simulink model "model_openloop"  (R2021a)
settings: Solver=VariableStepAuto  StartTime=0.0  StopTime=100  RelTol=1e-3  EnableMultiTasking=on
values from neighbouring files (symbols this model uses):
  BE_rpm2kgps = BE_rpm2mmps*BE_mm2cc*BE_cc2g/1000    (= 5.30929158457e-05)    [constants.m]
  Cnst = [jf1,jf2,jf3,jh1,jh2,jh3,mf1,mf2,mf3,mh,mp,rbx,m,g,kd0,kd,kl0,kl,km0,km,k1,k2]    [constants.m]
  mb0 = 1    [constants.m]
  MM_MM_rpms2mpss = MM_rpms2mmpss*MM_mm2mm/1000    (= 2.27603686636e-05)    [constants.m]
  RM_costet2z = 2    [constants.m]
  RM_rpm2radps = 2*pi/60    (= 0.10471975512)    [constants.m]
  RM_sintet2y = 2    [constants.m]
  rpx0 = 0    [constants.m]
  rpy0 = 0    [constants.m]
  rpz0 = 0.05    [constants.m]
settings Model: Creator=Zein  LastModifiedBy=zein
settings SolverCC: AlgebraicLoopSolver=TrustRegion
settings DataIOCC: ReturnWorkspaceOutputs=off
settings OptimizationCC: LifeSpan=inf
settings DebuggingCC: SFUnexpectedBacktrackingDiag=warning  SFNoUnconditionalDefaultTransitionDiag=warning  SFMachineParentedDataDiag=warning  ArithmeticOperatorsInVariantConditions=warning
settings SFSimCC: SimUseLocalCustomCode=off  CustomCodeUndefinedFunction=UseInterfaceOnly
settings RTWCC: RTWUseLocalCustomCode=off
settings CodeAppCC: StateflowObjectComments=on
settings GRTTargetCC: TargetLangStandard=C89/C90 (ANSI)
settings ConfigComp: CovMetricSettings=dw  CovSaveCumulativeToWorkspaceVar=on  CovSaveSingleToWorkspaceVar=on  CovExternalEMLEnable=off

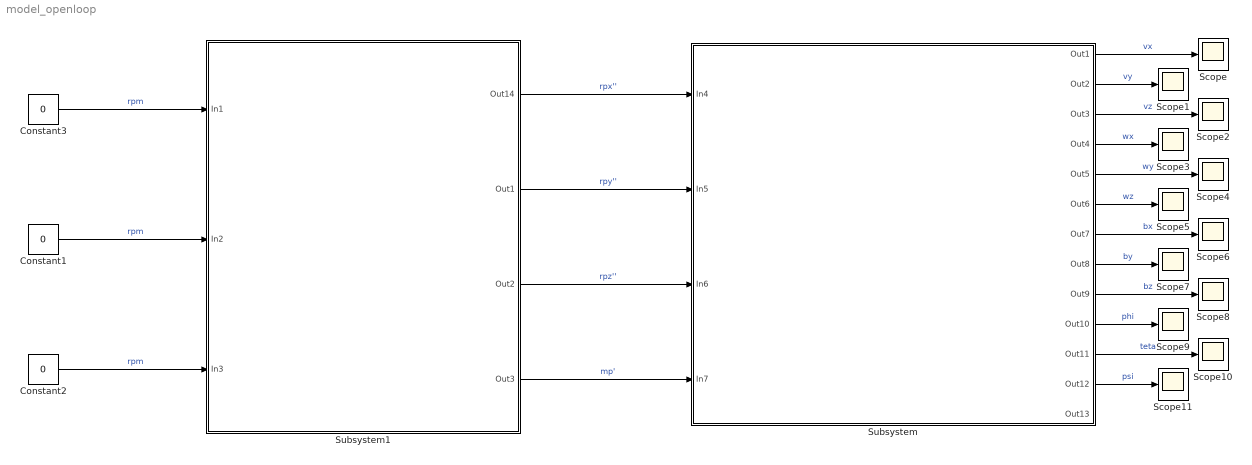
== system model_openloop ==
  Constant1 : Constant  Value=0
  Constant2 : Constant  Value=0
  Constant3 : Constant  Value=0
  Scope{,1..11} (12 alike) : Scope
  Subsystem : Subsystem
  Subsystem1 : Subsystem
  wires:
  Constant1/1 -> Subsystem1/2(In2)  "rpm"
  Constant2/1 -> Subsystem1/3(In3)  "rpm"
  Subsystem1/1(Out14) -> Subsystem/1(In4)  "rpx''"
  Subsystem1/2(Out1) -> Subsystem/2(In5)  "rpy''"
  Subsystem1/3(Out2) -> Subsystem/3(In6)  "rpz''"
  Subsystem1/4(Out3) -> Subsystem/4(In7)  "mp'"
  Subsystem/1(Out1) -> Scope/1  "vx"
  Subsystem/2(Out2) -> Scope1/1  "vy"
  Subsystem/4(Out4) -> Scope3/1  "wx"
  Subsystem/3(Out3) -> Scope2/1  "vz"
  Subsystem/6(Out6) -> Scope5/1  "wz"
  Subsystem/5(Out5) -> Scope4/1  "wy"
  Subsystem/7(Out7) -> Scope6/1  "bx"
  Subsystem/10(Out10) -> Scope9/1  "phi"
  Subsystem/9(Out9) -> Scope8/1  "bz"
  Subsystem/12(Out12) -> Scope11/1  "psi"
  Subsystem/11(Out11) -> Scope10/1  "teta"
  Subsystem/8(Out8) -> Scope7/1  "by"
  Constant3/1 -> Subsystem1/1(In1)  "rpm"

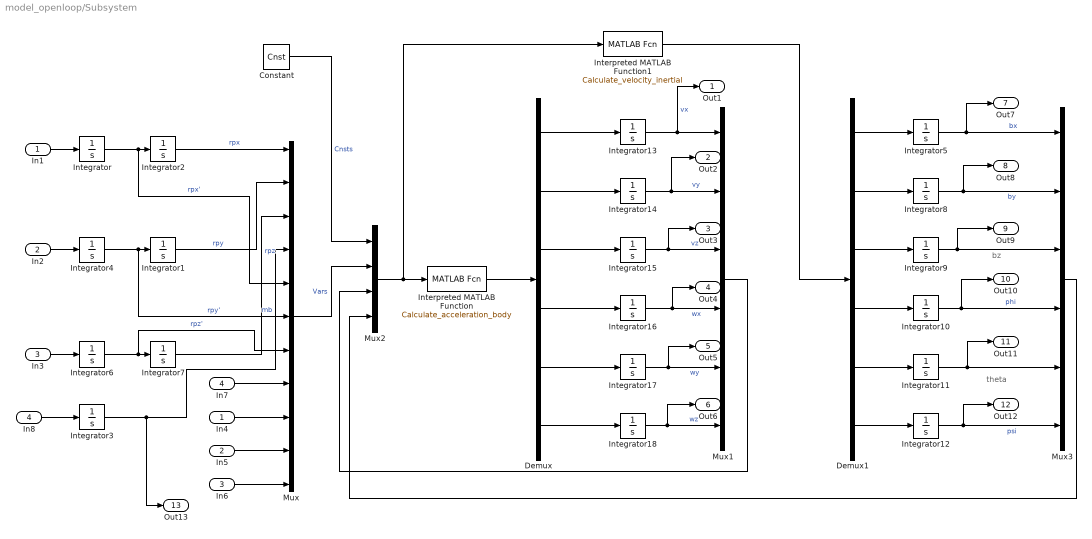
== system model_openloop/Subsystem ==
  note: theta
  note: bz
  In4 : Inport
  In5 : Inport  Port=2
  In6 : Inport  Port=3
  In7 : Inport  Port=4
  Constant : Constant  Value=Cnst
  Demux : Demux  Outputs=6
  Demux1 : Demux  Outputs=6
  In1 : InportShadow
  In2 : InportShadow  Port=2
  In3 : InportShadow  Port=3
  In8 : InportShadow  Port=4
  Integrator{,4..6,8..18} (15 alike) : Integrator
  Integrator1 : Integrator  InitialCondition=rpy0
  Integrator2 : Integrator  InitialCondition=rpx0
  Integrator3 : Integrator  InitialCondition=mb0
  Integrator7 : Integrator  InitialCondition=rpz0
  Interpreted MATLAB Function : MATLABFcn  MATLABFcn=Calculate_acceleration_body  OutputDimensions=6
  Interpreted MATLAB Function1 : MATLABFcn  MATLABFcn=Calculate_velocity_inertial  OutputDimensions=6  Output1D=off
  Mux : Mux  Inputs=11
  Mux1 : Mux  Inputs=6
  Mux2 : Mux
  Mux3 : Mux  Inputs=6
  Out1 : Outport
  Out2 : Outport  Port=2
  Out3 : Outport  Port=3
  Out4 : Outport  Port=4
  Out5 : Outport  Port=5
  Out6 : Outport  Port=6
  Out7 : Outport  Port=7
  Out8 : Outport  Port=8
  Out9 : Outport  Port=9
  Out10 : Outport  Port=10
  Out11 : Outport  Port=11
  Out12 : Outport  Port=12
  Out13 : Outport  Port=13
  wires:
  Demux1/2 -> Integrator8/1
  Integrator9/1 -> Out9/1, Mux3/3
  Integrator8/1 -> Out8/1, Mux3/2  "by"
  Integrator18/1 -> Out6/1, Mux1/6  "wz"
  Integrator16/1 -> Out4/1, Mux1/4  "wx"
  Demux/3 -> Integrator15/1
  Integrator15/1 -> Out3/1, Mux1/3  "vz"
  Interpreted MATLAB Function/1 -> Demux/1
  Demux/5 -> Integrator17/1
  Demux1/5 -> Integrator11/1
  Demux/2 -> Integrator14/1
  Mux3/1 -> Mux2/4
  Interpreted MATLAB Function1/1 -> Demux1/1
  Demux1/3 -> Integrator9/1
  Constant/1 -> Mux2/1  "Cnsts"
  Demux/6 -> Integrator18/1
  Demux/4 -> Integrator16/1
  Demux1/6 -> Integrator12/1
  Demux/1 -> Integrator13/1
  Integrator14/1 -> Out2/1, Mux1/2  "vy"
  Integrator17/1 -> Out5/1, Mux1/5  "wy"
  Demux1/4 -> Integrator10/1
  Integrator13/1 -> Out1/1, Mux1/1  "vx"
  Integrator12/1 -> Out12/1, Mux3/6  "psi"
  Integrator11/1 -> Out11/1, Mux3/5
  Integrator5/1 -> Out7/1, Mux3/1  "bx"
  Integrator10/1 -> Out10/1, Mux3/4  "phi"
  Demux1/1 -> Integrator5/1
  Mux2/1 -> Interpreted MATLAB Function1/1, Interpreted MATLAB Function/1
  Mux1/1 -> Mux2/3
  Integrator1/1 -> Mux/2  "rpy"
  Integrator/1 -> Mux/5, Integrator2/1  "rpx'"
  In6/1 -> Mux/11
  In5/1 -> Mux/10
  Integrator6/1 -> Mux/7, Integrator7/1  "rpz'"
  Integrator4/1 -> Mux/6, Integrator1/1  "rpy'"
  Integrator3/1 -> Out13/1, Mux/4  "mb"
  Integrator2/1 -> Mux/1  "rpx"
  Integrator7/1 -> Mux/3  "rpz"
  In7/1 -> Mux/8
  Mux/1 -> Mux2/2  "Vars"
  In4/1 -> Mux/9
  In1/1 -> Integrator/1
  In2/1 -> Integrator4/1
  In3/1 -> Integrator6/1
  In8/1 -> Integrator3/1

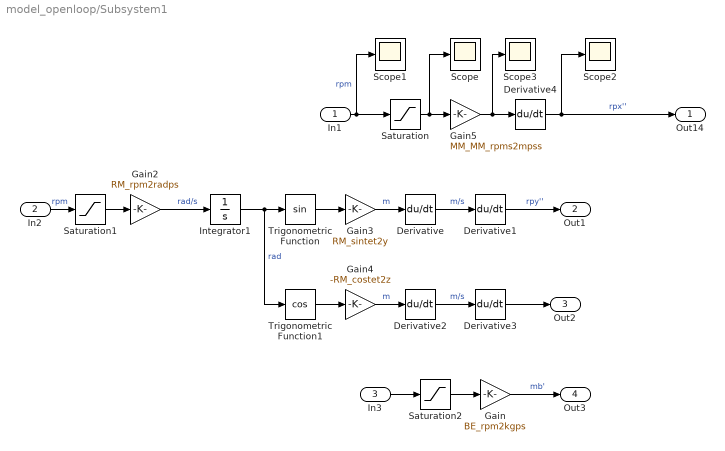
== system model_openloop/Subsystem1 ==
  In1 : Inport
  In2 : Inport  Port=2
  In3 : Inport  Port=3
  Derivative{,1..4} (5 alike) : Derivative
  Gain : Gain  Gain=BE_rpm2kgps
  Gain2 : Gain  Gain=RM_rpm2radps
  Gain3 : Gain  Gain=RM_sintet2y
  Gain4 : Gain  Gain=-RM_costet2z
  Gain5 : Gain  Gain=MM_MM_rpms2mpss
  Integrator1 : Integrator
  Saturation : Saturate  UpperLimit=350  LowerLimit=-350
  Saturation1 : Saturate  UpperLimit=350  LowerLimit=-350
  Saturation2 : Saturate  UpperLimit=350  LowerLimit=-350
  Scope{,1..3} (4 alike) : Scope
  Trigonometric Function : Trigonometry
  Trigonometric Function1 : Trigonometry  Operator=cos
  Out14 : Outport
  Out1 : Outport  Port=2
  Out2 : Outport  Port=3
  Out3 : Outport  Port=4
  wires:
  Derivative/1 -> Derivative1/1  "m/s"
  Derivative1/1 -> Out1/1  "rpy''"
  Gain4/1 -> Derivative2/1  "m"
  In3/1 -> Saturation2/1
  Derivative3/1 -> Out2/1
  Derivative4/1 -> Out14/1, Scope2/1  "rpx''"
  Derivative2/1 -> Derivative3/1  "m/s"
  Integrator1/1 -> Trigonometric Function1/1, Trigonometric Function/1  "rad"
  Trigonometric Function1/1 -> Gain4/1
  Trigonometric Function/1 -> Gain3/1
  Gain/1 -> Out3/1  "mb'"
  Gain2/1 -> Integrator1/1  "rad/s"
  Gain3/1 -> Derivative/1  "m"
  In1/1 -> Scope1/1, Saturation/1  "rpm"
  Saturation1/1 -> Gain2/1
  In2/1 -> Saturation1/1  "rpm"
  Saturation2/1 -> Gain/1
  Saturation/1 -> Scope/1, Gain5/1
  Gain5/1 -> Scope3/1, Derivative4/1
